simulink model "estimador_part5_v2"  (R2020a)
settings: Solver=VariableStepAuto  StartTime=0.0  StopTime=30  MaxStep=0.0005  RelTol=1e-3
values from neighbouring files (symbols this model uses):
  C = 1    [hugo_lab2_enviar.m]    (also in part_5.m = [eye(3),zeros(3)]; part_5_v2.m = [eye(3),zeros(3)]; sensor_properties.m)
  inputTs = 0.005    [part_5_v2.m]
  P0 = Q    [part_5_v2.m]
  Q = 1e-2    (= 0.01)    [hugo_lab2_enviar.m]    (also in part_5.m = diag([cov_w,cov_bias]); part_5_v2.m = diag([cov_w,cov_bias]); sensor_properties.m)
  R = 1e-1    (= 0.1)    [hugo_lab2_enviar.m]    (also in part_5.m = diag(cov_y); part_5_v2.m = diag(cov_y); sensor_properties.m)
  x0 = [y(1,2:4)';zeros(3,1)]    [part_5_v2.m]    (also in sensor_properties.m = [0 0])
settings Model: Creator=josea  LastModifiedBy=josem
settings DataIOCC: ReturnWorkspaceOutputs=off
settings DebuggingCC: ArithmeticOperatorsInVariantConditions=warning
settings SFSimCC: SimUseLocalCustomCode=off  CustomCodeUndefinedFunction=UseInterfaceOnly
settings RTWCC: RTWUseLocalCustomCode=off

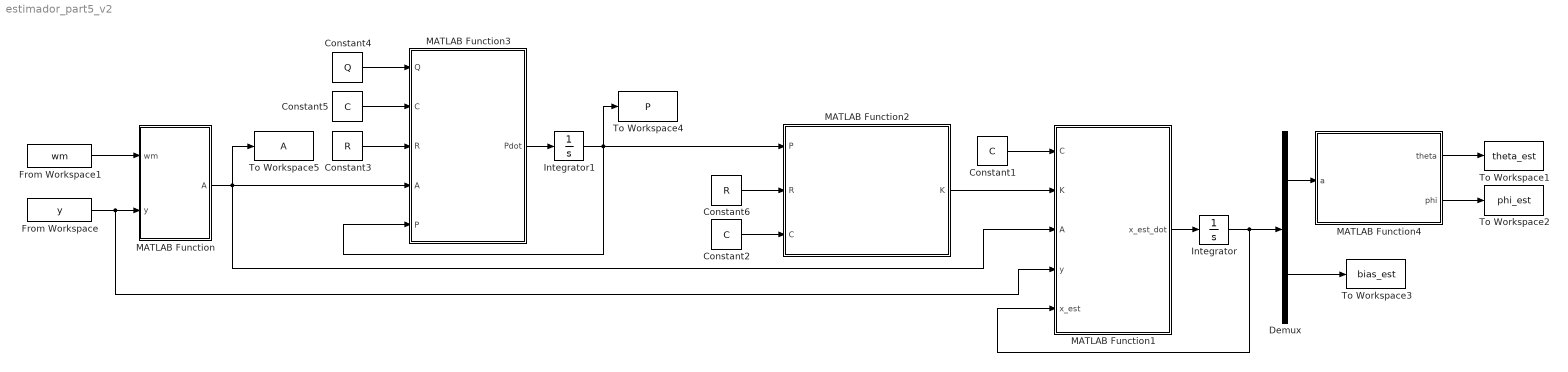
== system estimador_part5_v2 ==
  Constant1 : Constant  Value=C
  Constant2 : Constant  Value=C
  Constant3 : Constant  Value=R
  Constant4 : Constant  Value=Q
  Constant5 : Constant  Value=C
  Constant6 : Constant  Value=R
  Demux : Demux  Outputs=[3,3]
  From Workspace : FromWorkspace  VariableName=y  SampleTime=inputTs
  From Workspace1 : FromWorkspace  VariableName=wm  SampleTime=inputTs
  Integrator : Integrator  InitialCondition=x0
  Integrator1 : Integrator  InitialCondition=P0
  MATLAB Function : MATLAB Function  TreatAsAtomicUnit=on
  MATLAB Function1 : MATLAB Function  TreatAsAtomicUnit=on
  MATLAB Function2 : MATLAB Function  TreatAsAtomicUnit=on
  MATLAB Function3 : MATLAB Function  TreatAsAtomicUnit=on
  MATLAB Function4 : MATLAB Function  TreatAsAtomicUnit=on
  To Workspace1 : ToWorkspace  VariableName=theta_est  SaveFormat=Structure With Time  SampleTime=-1
  To Workspace2 : ToWorkspace  VariableName=phi_est  SaveFormat=Structure With Time  SampleTime=-1
  To Workspace3 : ToWorkspace  VariableName=bias_est  SaveFormat=Structure With Time  SampleTime=-1
  To Workspace4 : ToWorkspace  VariableName=P  SaveFormat=Structure With Time  SampleTime=-1
  To Workspace5 : ToWorkspace  VariableName=A  SaveFormat=Structure With Time  SampleTime=-1
  wires:
  From Workspace/1 -> MATLAB Function1/4(y), MATLAB Function/2(y)
  From Workspace1/1 -> MATLAB Function/1(wm)
  Integrator/1 -> MATLAB Function1/5(x_est), Demux/1
  MATLAB Function1/1(x_est_dot) -> Integrator/1
  Constant1/1 -> MATLAB Function1/1(C)
  MATLAB Function2/1(K) -> MATLAB Function1/2(K)
  Constant6/1 -> MATLAB Function2/2(R)
  MATLAB Function/1(A) -> MATLAB Function1/3(A), To Workspace5/1, MATLAB Function3/4(A)
  Constant2/1 -> MATLAB Function2/3(C)
  Integrator1/1 -> MATLAB Function2/1(P), To Workspace4/1, MATLAB Function3/5(P)
  MATLAB Function3/1(Pdot) -> Integrator1/1
  Constant3/1 -> MATLAB Function3/3(R)
  Constant5/1 -> MATLAB Function3/2(C)
  Constant4/1 -> MATLAB Function3/1(Q)
  Demux/1 -> MATLAB Function4/1(a)
  Demux/2 -> To Workspace3/1
  MATLAB Function4/2(phi) -> To Workspace2/1
  MATLAB Function4/1(theta) -> To Workspace1/1

== matlab function estimador_part5_v2/MATLAB Function1 ==
  data: C input; K input; A input; y input; x_est_dot output; x_est input
function x_est_dot = dynamics(C,K,A,y,x_est)
    x_est_dot = A*x_est+K*(y-C*x_est);
end

== matlab function estimador_part5_v2/MATLAB Function ==
  data: wm input; y input; A output
function A = createA(wm,y)
    Swm = skew(wm);
    Sy = skew(y);
    
    A = [-Swm,-Sy;
         zeros(3),zeros(3)];
end

function S = skew(v)
    S = [0, -v(3), v(2);
        v(3), 0, -v(1);
        -v(2), v(1), 0];
end

== matlab function estimador_part5_v2/MATLAB Function2 ==
  data: P input; R input; C input; K output
function K = createK(P,R,C)
    K = P*C'/R;
end

== matlab function estimador_part5_v2/MATLAB Function3 ==
  data: Q input; C input; R input; A input; Pdot output; P input
function Pdot = getPdot(Q,C,R,A,P)
    Pdot = A*P+P*A'+Q-P*C'/R*C*P;
end

== matlab function estimador_part5_v2/MATLAB Function4 ==
  data: a input; theta output; phi output
function [theta,phi] = calc_theta_phi(a)
    phi = 180/pi*atan(a(2)/a(3));
    theta = 180/pi*atan(a(1)/sqrt(a(2)^2 + a(3)^2));
end
